simulink model "AeroPlantMIACpart3"  (R2022b)
settings: Solver=ode45  StartTime=0.0  StopTime=100  RelTol=1e-3  EnableMultiTasking=on
values from neighbouring files (symbols this model uses):
  sigma2e = 0.0    (= 0)    [inpart3.m]
  Ta = 0.05    [inpart3.m]
  Tc = 0.001    [inpart3.m]
  TF = 1.5*Ta    (= 0.075)    [inpart3.m]
  wr = 0.25    [inpart3.m]
  Yr = 0.15    [inpart3.m]
libraries: simulink x1
settings Model: Creator=e.amutete  LastModifiedBy=ASUS
settings SolverCC: AlgebraicLoopSolver=TrustRegion
settings DataIOCC: LimitDataPoints=on  SaveFormat=Array  SignalLoggingSaveFormat=ModelDataLogs  ReturnWorkspaceOutputs=off
settings OptimizationCC: InitFltsAndDblsToZero=on  LifeSpan=inf
settings DebuggingCC: SaveWithParameterizedLinksMsg=none  UnderspecifiedInitializationDetection=Classic  MergeDetectMultiDrivingBlocksExec=none  SignalResolutionControl=TryResolveAllWithWarning  SolverPrmCheckMsg=warning  MultiTaskDSMMsg=warning  MultiTaskCondExecSysMsg=none  FcnCallInpInsideContextMsg=warning  UnconnectedInputMsg=warning  UnconnectedOutputMsg=warning  UnconnectedLineMsg=warning  SFUnexpectedBacktrackingDiag=warning  SFNoUnconditionalDefaultTransitionDiag=warning  SFExecutionAtInitializationDiag=none  SFMachineParentedDataDiag=warning  ArithmeticOperatorsInVariantConditions=warning
settings HardwareCC: ProdBitPerPointer=32  ProdBitPerSizeT=32  ProdBitPerPtrDiffT=32  ProdLargestAtomicFloat=None  ProdIntDivRoundTo=Undefined  ProdEndianess=Unspecified  ProdWordSize=32  ProdHWDeviceType=32-bit Generic
settings ModelReferenceCC: EnableRefExpFcnMdlSchedulingChecks=on  PropagateSignalLabelsOutOfModel=off
settings SFSimCC: SimUseLocalCustomCode=off  CustomCodeUndefinedFunction=UseInterfaceOnly
settings RTWCC: RTWUseLocalCustomCode=off
settings CodeAppCC: StateflowObjectComments=on
settings GRTTargetCC: TargetFcnLib=ansi_tfl_tmw.mat  TargetLangStandard=C89/C90 (ANSI)  CombineOutputUpdateFcns=off  GRTInterface=on
settings ConfigComp: CovMetricSettings=dw  CovSaveCumulativeToWorkspaceVar=on  CovSaveSingleToWorkspaceVar=on  CovExternalEMLEnable=off

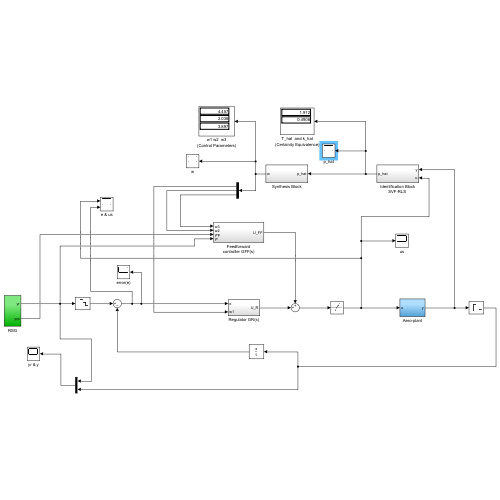
[thumbnail: Simulink's stored preview of the top-level diagram]
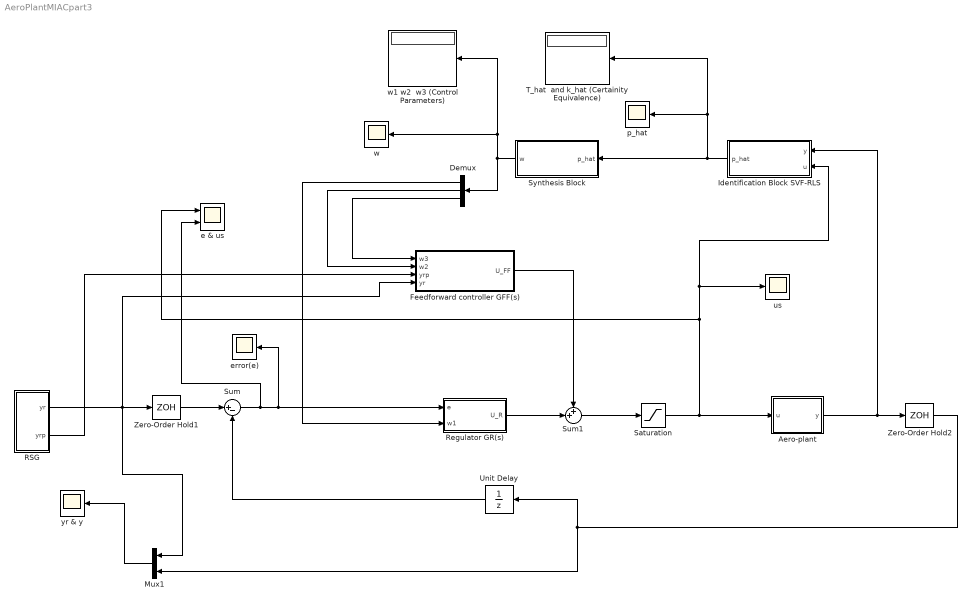
== system AeroPlantMIACpart3 ==
  Aero-plant : Subsystem
  Demux : Demux  Outputs=[1 1 1]
  Feedforward controller GFF(s) : Subsystem
  "Identification Block SVF-RLS " : Subsystem
  Mux1 : Mux  Inputs=2
  RSG : Subsystem
  Regulator GR(s) : Subsystem
  Saturation : Saturate  UpperLimit=pi  LowerLimit=-pi
  Sum : Sum  Inputs=|+-
  Sum1 : Sum  Inputs=++|
  Synthesis Block : Subsystem
  T_hat  and k_hat (Certainity Equivalence) : Display
  Unit Delay : UnitDelay  SampleTime=Tc  HasFrameUpgradeWarning=on
  Zero-Order Hold1 : ZeroOrderHold  SampleTime=Tc
  Zero-Order Hold2 : ZeroOrderHold  SampleTime=Tc
  e & us : Scope  NumInputPorts=2
  error(e) : Scope
  p_hat : Scope
  us : Scope
  w : Scope
  w1 w2  w3 (Control Parameters) : Display
  yr & y : Scope
  wires:
  RSG/1(yr) -> Mux1/1, Zero-Order Hold1/1, Feedforward controller GFF(s)/4(yr)
  "Identification Block SVF-RLS "/1(p_hat) -> Synthesis Block/1(p_hat), T_hat  and k_hat (Certainity Equivalence)/1, p_hat/1
  Synthesis Block/1(w) -> w1 w2  w3 (Control Parameters)/1, w/1, Demux/1
  Unit Delay/1 -> Sum/2
  Sum/1 -> e & us/2, Regulator GR(s)/1(e), error(e)/1
  Feedforward controller GFF(s)/1(U_FF) -> Sum1/1
  Regulator GR(s)/1(U_R) -> Sum1/2
  Aero-plant/1(y) -> Zero-Order Hold2/1, "Identification Block SVF-RLS "/1(y)
  Zero-Order Hold1/1 -> Sum/1
  Demux/1 -> Regulator GR(s)/2(w1)
  Demux/2 -> Feedforward controller GFF(s)/2(w2)
  Demux/3 -> Feedforward controller GFF(s)/1(w3)
  RSG/2(yrp) -> Feedforward controller GFF(s)/3(yrp)
  Mux1/1 -> yr & y/1
  Zero-Order Hold2/1 -> Mux1/2, Unit Delay/1
  Sum1/1 -> Saturation/1
  Saturation/1 -> e & us/1, "Identification Block SVF-RLS "/2(u), us/1, Aero-plant/1(u)

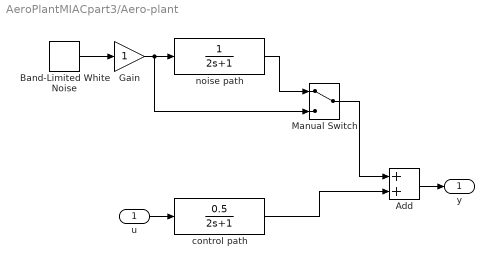
== system AeroPlantMIACpart3/Aero-plant ==
  u : Inport
  Add : Sum
  Band-Limited White Noise : simulink/Sources/Band-Limited White Noise  Cov=[sigma2e*Tc]  Ts=Tc  seed=[23341]
  Gain : Gain
  Manual Switch : ManualSwitch
  control path : TransferFcn  Numerator=[0.5]  Denominator=[2 1]
  noise path : TransferFcn  Denominator=[2 1]
  y : Outport
  wires:
  control path/1 -> Add/2
  Band-Limited White Noise/1 -> Gain/1
  Gain/1 -> Manual Switch/2, noise path/1
  Add/1 -> y/1
  u/1 -> control path/1
  noise path/1 -> Manual Switch/1
  Manual Switch/1 -> Add/1

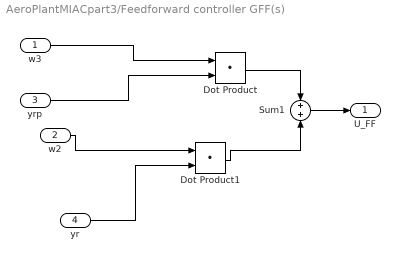
== system AeroPlantMIACpart3/Feedforward controller GFF(s) ==
  w3 : Inport
  w2 : Inport  Port=2
  yrp : Inport  Port=3
  yr : Inport  Port=4
  Dot Product : DotProduct  OutDataTypeStr=Inherit: Inherit via internal rule
  Dot Product1 : DotProduct  OutDataTypeStr=Inherit: Inherit via internal rule
  Sum1 : Sum
  U_FF : Outport
  wires:
  w2/1 -> Dot Product1/1
  Dot Product/1 -> Sum1/1
  Dot Product1/1 -> Sum1/2
  Sum1/1 -> U_FF/1
  yr/1 -> Dot Product1/2
  yrp/1 -> Dot Product/2
  w3/1 -> Dot Product/1

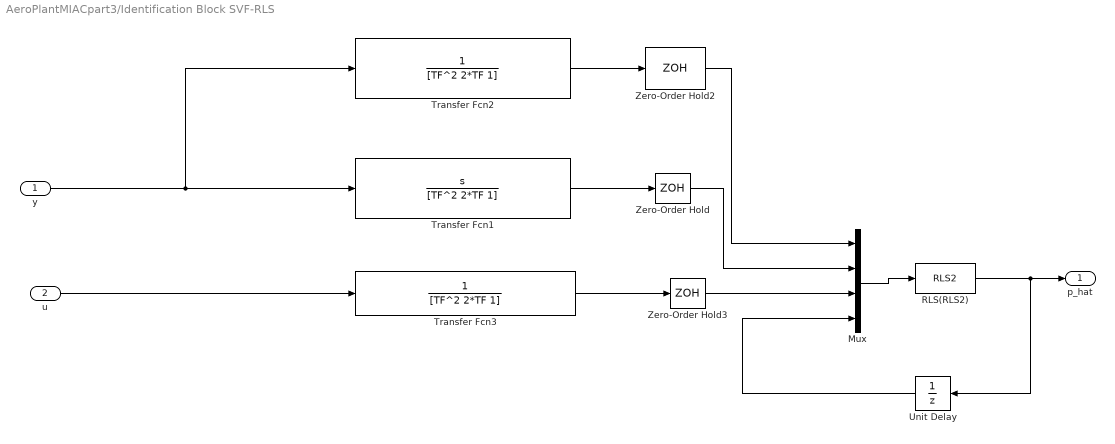
== system AeroPlantMIACpart3/Identification Block SVF-RLS  ==
  y : Inport
  u : Inport  Port=2
  Mux : Mux
  RLS(RLS2) : MATLABFcn  MATLABFcn=RLS2  SampleTime=Ta
  Transfer Fcn1 : TransferFcn  Numerator=[1 0]  Denominator=[TF^2 2*TF 1]
  Transfer Fcn2 : TransferFcn  Denominator=[TF^2 2*TF 1]
  Transfer Fcn3 : TransferFcn  Numerator=[1 ]  Denominator=[TF^2 2*TF 1]
  Unit Delay : UnitDelay  SampleTime=-1  HasFrameUpgradeWarning=on
  Zero-Order Hold : ZeroOrderHold  SampleTime=Ta
  Zero-Order Hold2 : ZeroOrderHold  SampleTime=Ta
  Zero-Order Hold3 : ZeroOrderHold  SampleTime=Ta
  p_hat : Outport
  wires:
  Transfer Fcn1/1 -> Zero-Order Hold/1
  Transfer Fcn2/1 -> Zero-Order Hold2/1
  Zero-Order Hold2/1 -> Mux/1
  Zero-Order Hold/1 -> Mux/2
  Mux/1 -> RLS(RLS2)/1
  RLS(RLS2)/1 -> p_hat/1, Unit Delay/1
  y/1 -> Transfer Fcn1/1, Transfer Fcn2/1
  u/1 -> Transfer Fcn3/1
  Transfer Fcn3/1 -> Zero-Order Hold3/1
  Zero-Order Hold3/1 -> Mux/3
  Unit Delay/1 -> Mux/4

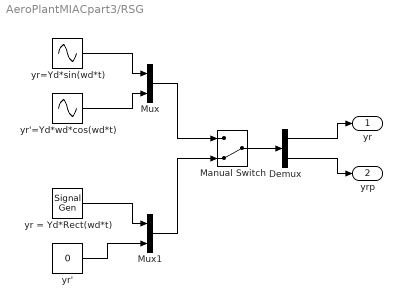
== system AeroPlantMIACpart3/RSG ==
  Demux : Demux  Outputs=2
  Manual Switch : ManualSwitch  CurrentSetting=0
  Mux : Mux  Inputs=2
  Mux1 : Mux  Inputs=2
  yr = Yd*Rect(wd*t) : SignalGenerator  WaveForm=square  Amplitude=Yr  Frequency=wr  Units=rad/sec
  yr' : Constant  Value=0
  yr'=Yd*wd*cos(wd*t) : Sin  Amplitude=Yr*wr  Frequency=wr  Phase=pi/2  SampleTime=0
  yr=Yd*sin(wd*t) : Sin  Amplitude=Yr  Frequency=wr  SampleTime=0
  yr : Outport
  yrp : Outport  Port=2
  wires:
  yr=Yd*sin(wd*t)/1 -> Mux/1
  yr'=Yd*wd*cos(wd*t)/1 -> Mux/2
  yr = Yd*Rect(wd*t)/1 -> Mux1/1
  yr'/1 -> Mux1/2
  Mux/1 -> Manual Switch/1
  Mux1/1 -> Manual Switch/2
  Manual Switch/1 -> Demux/1
  Demux/1 -> yr/1
  Demux/2 -> yrp/1

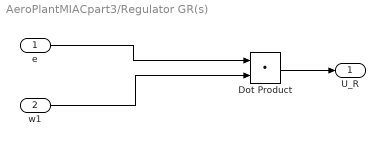
== system AeroPlantMIACpart3/Regulator GR(s) ==
  e : Inport
  w1 : Inport  Port=2
  Dot Product : DotProduct  OutDataTypeStr=Inherit: Inherit via internal rule
  U_R : Outport
  wires:
  e/1 -> Dot Product/1
  Dot Product/1 -> U_R/1
  w1/1 -> Dot Product/2

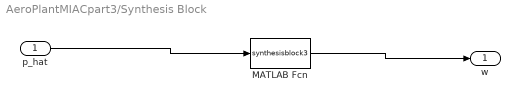
== system AeroPlantMIACpart3/Synthesis Block ==
  p_hat : Inport
  MATLAB Fcn : MATLABFcn  MATLABFcn=synthesisblock3  SampleTime=Ta
  w : Outport
  wires:
  p_hat/1 -> MATLAB Fcn/1
  MATLAB Fcn/1 -> w/1
